simulink model "model_AllInOne1 (1)"  (R2013a)
settings: Solver=ode45  StartTime=0.0  StopTime=400  RelTol=1e-3
undefined symbols (not defined in the file or in its folder): generateDummyBeams, m, s
libraries: test_library x15, aerolib6dofsys x2, aerolibtransform2 x1, aerolibutil x1, aerolibconvert2 x1, falter_library x1, vrlib x1
(part 1 of 2)
settings Model: Creator=elm  LastModifiedBy=alim
settings DataIOCC: SignalLoggingSaveFormat=ModelDataLogs  SaveOutput=off  SignalLogging=off  DSMLogging=off  SaveTime=off
settings OptimizationCC: ExpressionDepthLimit=2147483647  EfficientMapNaN2IntZero=off
settings DebuggingCC: FcnCallInpInsideContextMsg=UseLocalSettings
settings HardwareCC: TargetBitPerLong=64  TargetBitPerPointer=64  TargetIntDivRoundTo=Zero  TargetEndianess=LittleEndian  TargetWordSize=64  TargetHWDeviceType=MATLAB Host  ProdEqTarget=off
settings SFSimCC: SimParseCustomCode=off
settings CodeAppCC: MaxIdLength=128
settings GRTTargetCC: CombineOutputUpdateFcns=off  GRTInterface=on

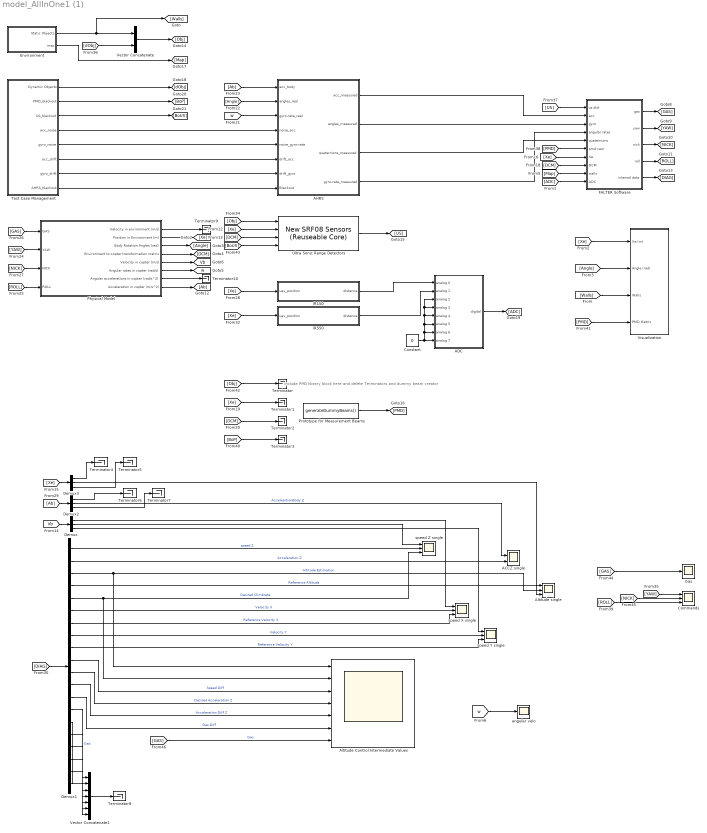
== system model_AllInOne1 (1) ==
  note: include PMD library block  here and delete Terminators
      | and dummy beam creator
  ACCZ single : Scope  NumInputPorts=2
      settings: ShowLegends=on  TimeRange=5  YMin=-9.9~9.7331  YMax=-8.7~9.7343  SaveName=ScopeData4  SampleInput=on
  ADC : Subsystem
  AHRS : Subsystem
  Altitude Control Intermediate Values : Scope  NumInputPorts=7
      settings: ShowLegends=on  TimeRange=20  YMin=0.1~-0.2~-0.9~-0.5~-0.4~-0.00015~0  YMax=1.3~0.5~0.5~0.3~0.3~0.00015~150  SaveName=ScopeData16  SampleInput=on
  Altitude single : Scope  NumInputPorts=3
      settings: TimeRange=15  YMin=0.1~0.1~0  YMax=1.3~1.3~1  SaveName=ScopeData7  SampleInput=on
  Commands : Scope  NumInputPorts=3
      settings: YMin=0~0.1~0  YMax=3.25~0.8~1  SaveName=ScopeData32  SampleInput=on
  Constant : Constant  Value=0
  Demux : Demux  Outputs=3
  Demux1 : Demux  Outputs=20
  Demux2 : Demux  Outputs=3
  Demux3 : Demux  Outputs=3
  Environment : Subsystem
  FALTER Software : Subsystem
  Gas : Scope
      settings: TimeRange=18  YMin=0  YMax=300  SaveName=ScopeData31  SampleInput=on
  IR150 : Subsystem
  IR550 : Subsystem
  Physical Model : Subsystem
  Prototype for Measurement Beams : Constant  Value=generateDummyBeams()  OutDataTypeStr=single
  Terminator{,1..10} (11 alike) : Terminator
  Test Case Management : Subsystem
  "Ultra Sonic Range Detectors " : falter_library/New SRF08 Sensors  (Reuseable Core)  a=[0.1 0 0 0 -1 0; 0 0.12 -0.07 0 -1 0; 0 0.12 0.07 0 0 1; 0 0 0.21 1 0 0; 0.07 0.12 0 1 0 0; 0 0 -0.21 1 0 0; -0.07 0.12 0 -1 0 0; 0 0.12 0 0 1 0]  t=0.05
  Vector Concatenate : Concatenate  Mode=Multidimensional array
  Vector Concatenate1 : Concatenate  NumInputs=7  Mode=Multidimensional array
  Visualization : Subsystem
  angular velo : Scope
      settings: TimeRange=7.5  YMin=-0.85  YMax=0  SaveName=ScopeData24  SampleInput=on
  speed X single : Scope  NumInputPorts=3
      settings: TimeRange=5  YMin=-0.05~-0.025~0  YMax=0.175~0.15~0.3  SaveName=ScopeData14  SampleInput=on
  speed Y single : Scope  NumInputPorts=3
      settings: YMin=0~-5~-5  YMax=10~5~5  SaveName=ScopeData25  SampleInput=on
  speed Z single : Scope  NumInputPorts=3
      settings: TimeRange=18  YMin=-5~-5~-0.2  YMax=5~5~0.2  SaveName=ScopeData5  SampleInput=on
  tag scope: Vb=global, w=global
  wires:
  [Walls] -> Visualization/3(Walls)
  [Xe] -> Visualization/1(Xe (m))
  [Angle] -> Visualization/2(Angle (rad))
  Environment/1(Static Objects) -> Vector Concatenate/1, [Walls]
  FALTER Software/1(gas) -> [GAS]
  FALTER Software/2("yaw ") -> [YAW]
  FALTER Software/3(nick) -> [NICK]
  FALTER Software/4(roll) -> [ROLL]
  Physical Model/1(Velocity in environment (m/s)) -> Terminator9/1
  Physical Model/2(Position in Environment (m)) -> [Xe]
  [Xe] -> "Ultra Sonic Range Detectors "/2
  Physical Model/7(Angular accelerations in copter (rad/s^2)) -> Terminator10/1
  Physical Model/5(Velocity in copter (m/s)) -> [Vb]
  Physical Model/4(Environment to copter transformation matrix) -> [DCM]
  Physical Model/3(Body Rotation Angles (rad)) -> [Angle]
  Physical Model/8(Acceleration in copter (m/s^2)) -> [Ab]
  [YAW] -> Physical Model/2(YAW)
  [NICK] -> Physical Model/3(NICK)
  [ROLL] -> Physical Model/4(ROLL)
  [DCM] -> "Ultra Sonic Range Detectors "/3
  Vector Concatenate/1 -> [Obj]
  [Obj] -> Terminator/1
  FALTER Software/5(internal data) -> [DIAG]
  Test Case Management/1(Dynamic Objects) -> [dObj]
  [PMD] -> Visualization/4(PMD Matrix)
  [Obj] -> "Ultra Sonic Range Detectors "/1
  [dObj] -> Vector Concatenate/2
  Test Case Management/3(US_blackout) -> [BoUS]
  Test Case Management/2(PMD_blackout) -> [BoP]
  [BoUS] -> "Ultra Sonic Range Detectors "/4
  "Ultra Sonic Range Detectors "/1 -> [US]
  [DIAG] -> Demux1/1
  [Ab] -> Demux2/1
  Demux1/9 -> speed Y single/3  "Reference Velocity Y"
  Demux1/7 -> speed X single/3  "Reference Velocity X"
  Demux1/8 -> speed Y single/2  "Velocity Y"
  [Xe] -> Demux3/1
  [Vb] -> Demux/1
  Demux1/1 -> speed Z single/2  "speed Z"
  Demux1/3 -> Altitude single/2, Altitude Control Intermediate Values/1  "Altitude Estimation"
  Demux1/4 -> Altitude single/3  "Reference Altitude"
  Demux1/2 -> ACCZ single/2  "Acceleration Z"
  Demux/2 -> speed Z single/1
  Demux1/6 -> speed X single/2  "Velocity X"
  Demux1/5 -> speed Z single/3, Altitude Control Intermediate Values/2  "Desired Climbrate"
  Demux/1 -> speed X single/1
  Demux/3 -> speed Y single/1
  Demux2/2 -> ACCZ single/1  "AcceleartionBody Z"
  Demux3/2 -> Altitude single/1
  [Xe] -> IR150/1(uav_position)
  [Xe] -> IR550/1(uav_position)
  [GAS] -> Gas/1
  [YAW] -> Commands/1
  [NICK] -> Commands/2
  [ROLL] -> Commands/3
  [GAS] -> Physical Model/1(GAS)
  Demux1/10 -> Altitude Control Intermediate Values/3  "Speed Diff"
  Demux1/11 -> Altitude Control Intermediate Values/4  "Desired Acceleration Z"
  Demux1/12 -> Altitude Control Intermediate Values/5  "Acceleration Diff Z"
  Demux1/13 -> Altitude Control Intermediate Values/6  "Gas Diff"
  [GAS] -> Altitude Control Intermediate Values/7  "Gas"
  Prototype for Measurement Beams/1 -> [PMD]
  [Xe] -> Terminator1/1
  [DCM] -> Terminator2/1
  [BoP] -> Terminator3/1
  Demux3/1 -> Terminator4/1
  Demux3/3 -> Terminator5/1
  Demux2/1 -> Terminator6/1
  Demux2/3 -> Terminator7/1
  Demux1/14 -> Vector Concatenate1/1  "Gas"
  Demux1/15 -> Vector Concatenate1/2
  Demux1/16 -> Vector Concatenate1/3
  Demux1/17 -> Vector Concatenate1/4
  Demux1/18 -> Vector Concatenate1/5
  Demux1/19 -> Vector Concatenate1/6
  Demux1/20 -> Vector Concatenate1/7
  Vector Concatenate1/1 -> Terminator8/1
  Environment/2(map) -> [Map]
  Physical Model/6(Angular rates in copter (rad/s)) -> [w]
  [w] -> angular velo/1
  ADC/1(digital) -> [ADC]
  [w] -> AHRS/3(gyro-rate_real)
  [Angle] -> AHRS/2(angles_real)
  [Ab] -> AHRS/1(acc_body)
  Test Case Management/8(AHRS_blackout) -> AHRS/8(Blackout)
  Test Case Management/7(gyro_drift) -> AHRS/7(drift_gyro)
  Test Case Management/6(acc_drift) -> AHRS/6(drift_acc)
  Test Case Management/5(gyro_noise) -> AHRS/5(noise_gyro-rate)
  Test Case Management/4(acc_noise) -> AHRS/4(noise_acc)
  AHRS/2(angles_measured) -> FALTER Software/3(gyro)
  [US] -> FALTER Software/1(us dist)
  AHRS/1(acc_measured) -> FALTER Software/2(acc)
  AHRS/3(quaternions_measured) -> FALTER Software/5(quaternions)
  AHRS/4(gyro-rate_measured) -> FALTER Software/4(angular rates)
  [PMD] -> FALTER Software/6(pmd cam)
  [Xe] -> FALTER Software/7(Xe)
  [DCM] -> FALTER Software/8(DCM)
  [Map] -> FALTER Software/9(walls)
  [ADC] -> FALTER Software/10(ADC)
  Constant/1 -> ADC/6(analog 5), ADC/5(analog 4), ADC/3(analog 2), ADC/4(analog 3), ADC/7(analog 6), ADC/8(analog 7)
  IR150/1(distance) -> ADC/1(analog 0)
  IR550/1(distance) -> ADC/2(analog 1)

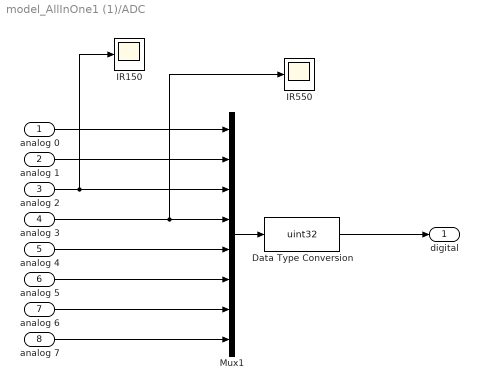
== system model_AllInOne1 (1)/ADC ==
  analog 0 : Inport
  analog 1 : Inport  Port=2
  analog 2 : Inport  Port=3
  analog 3 : Inport  Port=4
  analog 4 : Inport  Port=5
  analog 5 : Inport  Port=6
  analog 6 : Inport  Port=7
  analog 7 : Inport  Port=8
  Data Type Conversion : DataTypeConversion  OutMin=0  OutMax=1023  OutDataTypeStr=uint32
  IR150 : Scope
      settings: TimeRange=7.5  YMin=-0.85  YMax=0  SaveName=ScopeData9  SampleInput=on
  IR550 : Scope
      settings: TimeRange=7.5  YMin=-0.85  YMax=0  SaveName=ScopeData6  SampleInput=on
  Mux1 : Mux  Inputs=8
  digital : Outport
  wires:
  analog 0/1 -> Mux1/1
  analog 1/1 -> Mux1/2
  analog 2/1 -> Mux1/3, IR150/1
  analog 3/1 -> Mux1/4, IR550/1
  analog 4/1 -> Mux1/5
  analog 5/1 -> Mux1/6
  analog 6/1 -> Mux1/7
  analog 7/1 -> Mux1/8
  Mux1/1 -> Data Type Conversion/1
  Data Type Conversion/1 -> digital/1

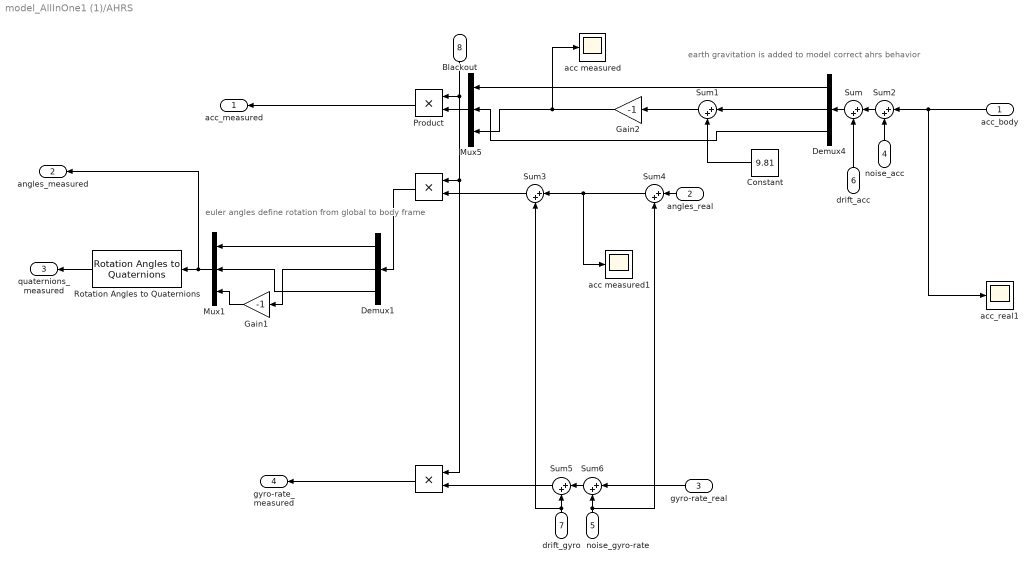
== system model_AllInOne1 (1)/AHRS ==
  note: earth gravitation is added to model correct
      | ahrs behavior
  note: euler angles define rotation
      | from global to body frame
  acc_body : Inport
  angles_real : Inport  Port=2
  gyro-rate_real : Inport  Port=3
  noise_acc : Inport  Port=4
  noise_gyro-rate : Inport  Port=5
  drift_acc : Inport  Port=6
  drift_gyro : Inport  Port=7
  Blackout : Inport  Port=8
  " " : Product  RndMeth=Zero
  "   " : Product  RndMeth=Zero
  Constant : Constant  Value=9.81
  Demux1 : Demux  Outputs=3
  Demux4 : Demux  Outputs=3
  Gain1 : Gain  Gain=-1
  Gain2 : Gain  Gain=-1
  Mux1 : Mux  Inputs=3
  Mux5 : Mux  Inputs=3
  Product : Product  RndMeth=Zero
  Rotation Angles to Quaternions : aerolibtransform2/Rotation Angles to Quaternions  rotationOrder=XYZ
  Sum{,1..6} (7 alike) : Sum  Inputs=|++
  acc measured : Scope
      settings: TimeRange=7.5  YMin=-11  YMax=-5  SampleInput=on
  acc measured1 : Scope
      settings: TimeRange=7.5  YMin=-11  YMax=-5  SaveName=ScopeData18  SampleInput=on
  acc_real1 : Scope
      settings: TimeRange=7.5  YMin=-0.85  YMax=0  SampleInput=on
  acc_measured : Outport
  angles_measured : Outport  Port=2
  quaternions_measured : Outport  Port=3
  gyro-rate_measured : Outport  Port=4
  wires:
  Demux4/1 -> Mux5/1
  " "/1 -> Demux1/1
  Sum/1 -> Demux4/1
  Sum2/1 -> Sum/1
  acc_body/1 -> Sum2/1, acc_real1/1
  noise_acc/1 -> Sum2/2
  drift_acc/1 -> Sum/2
  Mux5/1 -> Product/2
  Blackout/1 -> Product/1, " "/1, "   "/1
  Product/1 -> acc_measured/1
  Sum4/1 -> Sum3/1, acc measured1/1
  Sum3/1 -> " "/2
  angles_real/1 -> Sum4/1
  Sum6/1 -> Sum5/1
  "   "/1 -> gyro-rate_measured/1
  Sum5/1 -> "   "/2
  gyro-rate_real/1 -> Sum6/1
  drift_gyro/1 -> Sum5/2, Sum3/2
  noise_gyro-rate/1 -> Sum4/2, Sum6/2
  Rotation Angles to Quaternions/1 -> quaternions_measured/1
  Mux1/1 -> Rotation Angles to Quaternions/1, angles_measured/1
  Demux1/1 -> Mux1/1
  Demux4/2 -> Sum1/1
  Sum1/1 -> Gain2/1
  Constant/1 -> Sum1/2
  Gain2/1 -> Mux5/3, acc measured/1
  Demux4/3 -> Mux5/2
  Gain1/1 -> Mux1/3
  Demux1/3 -> Mux1/2
  Demux1/2 -> Gain1/1

== system model_AllInOne1 (1)/Environment ==
  note: basic walls for particle filter
  Terminator9 : Terminator
  environment model : Constant  RequirementInfo={}  Value=|
      | [
      |    -28     0   -16    10     0     0     0     0    32;
      |    -18     0    -5    36     0     0     0     0    10;
      |     18     0   -16    10     0     0     0     0    32;
      |     15     0     1     0     2     0     3     0     0;
      |      8     0     1     0     2     0     6     0     0;
      |      4     0     1     0     2     0     3     0     0;
      |      1     0     1     0     2     0     2     0     0;
      |     -2     0     1     0     2     0     2     0     0;
      |     -5     0     1     0     2     0     2     0     0;
      |     -8     0     1     0     2     0     3     0     0;
      |    -16     0     1     0     2     0     6     0     0;
      |    -18     0     1     0     2     0     1     0     0;
      |     15     0    -1     0     2     0     3     0     0;
      |      8     0    -1     0     2     0     6     0     0;
      |      4     0    -1     0     2     0     3     0     0;
      |      1     0    -1     0     2     0     2     0     0;
      |     -2     0    -1     0     2     0     2     0     0;
      |     -5     0    -1     0     2     0     2     0     0;
      |     -9     0    -1     0     2     0     3     0     0;
      |    -16     0    -1     0     2     0     6     0     0;
      |    -18     0    -1     0     2     0     1     0     0;
      |     10     0     5     0     2     0     0     0    -4;
      |      5     0     5     0     2     0     0     0    -4;
      |      2     0     5     0     2     0     0     0    -4;
      |     -1     0     5     0     2     0     0     0    -4;
      |     -4     0     5     0     2     0     0     0    -4;
      |     -7     0     5     0     2     0     0     0    -4;
      |    -12     0     5     0     2     0     0     0    -4;
      |     10     0    -5     0     2     0     0     0     4;
      |      5     0    -5     0     2     0     0     0     4,
      |      2     0    -5     0     2     0     0     0     4;
      |     -1     0    -5     0     2     0     0     0     4;
      |     -4     0    -5     0     2     0     0     0     4;
      |     -7     0    -5     0     2     0     0     0     4;
      |    -12     0    -5     0     2     0     0     0     4;
      |    -18     0     5     0     2     0    36     0     0;
      |    -18     0    -5     0     2     0    36     0     0;
      |     22     0   -11     0     2     0     0     0    -5;
      |     22     0    -8     0     2     0     0     0    -2;
      |     22     0    -5     0     2     0     0     0    -2;
      |     22     0    -1     0     2     0     0     0    -3;
      |     22     0     6     0     2     0     0     0    -5;
      |     22     0     8     0     2     0     0     0    -1;
      |     22     0    11     0     2     0     0     0    -2;
      |     22     0    16     0     2     0     0     0    -4;
      |     18     0    -9     0     2     0     4     0     0;
      |     18     0    -5     0     2     0     4     0     0;
      |     18     0    -1     0     2     0     4     0     0;
      |     18     0     1     0     2     0     4     0     0;
      |     18     0     7     0     2     0     4     0     0;
      |     18     0     9     0     2     0     4     0     0;
      |    -22     0   -11     0     2     0     0     0    -5;
      |    -22     0    -8     0     2     0     0     0    -2;
      |    -22     0    -5     0     2     0     0     0    -2;
      |    -22     0    -1     0     2     0     0     0    -3;
      |    -22     0     6     0     2     0     0     0    -5;
      |    -22     0     8     0     2     0     0     0    -1;
      |    -22     0    11     0     2     0     0     0    -2;
      |    -22     0    16     0     2     0     0     0    -4;
      |    -18     0    16     0     2     0     0     0   -15;
      |     18     0    16     0     2     0     0     0   -15;
      |     18     0   -16     0     2     0     0     0    15;
      |    -18     0   -16     0     2     0     0     0    15;
      |    -18     0    -9     0     2     0    -4     0     0;
      |    -18     0    -5     0     2     0    -4     0     0;
      |    -18     0    -1     0     2     0    -4     0     0;
      |    -18     0     1     0     2     0    -4     0     0;
      |    -18     0     7     0     2     0    -4     0     0;
      |    -18     0     9     0     2     0    -4     0     0;
      |     24     0   -14     0     2     0     0     0    -2;
      |     24     0    -6     0     2     0     0     0    -5;
      |     24     0    -4     0     2     0     0     0    -1;
      |     24     0    -1     0     2     0     0     0    -2;
      |     24     0     3     0     2     0     0     0    -2;
      |     24     0     5     0     2     0     0     0    -1;
      |     24     0    11     0     2     0     0     0    -5;
      |     24     0    16     0     2     0     0     0    -3;
      |     28     0   -12     0     2     0    -4     0     0;
      |     28     0    -8     0     2     0    -4     0     0;
      |     28     0    -5     0     2     0    -4     0     0;
      |     28     0    -1     0     2     0    -4     0     0;
      |     28     0     1     0     2     0    -4     0     0;
      |     28     0     5     0     2     0    -4     0     0;
      |     28     0     8     0     2     0    -4     0     0;
      |     28     0    12     0     2     0    -4     0     0;
      |    -24     0   -14     0     2     0     0     0    -2;
      |    -24     0    -6     0     2     0     0     0    -5;
      |    -24     0    -4     0     2     0     0     0    -1;
      |    -24     0    -1     0     2     0     0     0    -2;
      |    -24     0     3     0     2     0     0     0    -2;
      |    -24     0     5     0     2     0     0     0    -1;
      |    -24     0    11     0     2     0     0     0    -5;
      |    -24     0    16     0     2     0     0     0    -3;
      |    -28     0   -12     0     2     0     4     0     0;
      |    -28     0    -8     0     2     0     4     0     0;
      |    -28     0    -5     0     2     0     4     0     0;
      |    -28     0    -1     0     2     0     4     0     0;
      |    -28     0     1     0     2     0     4     0     0;
      |    -28     0     5     0     2     0     4     0     0;
      |    -28     0     8     0     2     0     4     0     0;
      |    -28     0    12     0     2     0     4     0     0;
      |    -28     0   -16     0     2     0    10     0     0;
      |    -28     0    16     0     2     0    10     0     0;
      |     28     0    16     0     2     0   -10     0     0;
      |     28     0   -16     0     2     0   -10     0     0;
      |     28     0   -16     0     2     0     0     0    32;
      |    -28     0   -16     0     2     0     0     0    32;
      | ]
  environment model1 : Constant  RequirementInfo={} %GIDa_a9006805_dc84_4529_b501_c6e675685754  Value=|
      | [
      |    -28     0   -16    10     0     0     0     0    32;
      |    -18     0    -5    36     0     0     0     0    10;
      |     18     0   -16    10     0     0     0     0    32;
      |    -24     0     1     0     2     0    -4     0     0;
      |    -24     0    -1     0     2     0    -4     0     0;
      |    -24     0    -1     0     2     0     0     0   -15;
      |    -22     0    -1     0     2     0     0     0   -15;
      |    -24     0     1     0     2     0     0     0    15;
      |    -22     0     1     0     2     0     0     0    15;
      |     22     0     1     0     2     0   -44     0     0;
      |     22     0    -1     0     2     0   -44     0     0;
      |     22     0    -1     0     2     0     0     0   -15;
      |     24     0    -1     0     2     0     0     0   -15;
      |     24     0    -1     0     2     0     4     0     0;
      |     24     0     1     0     2     0     4     0     0;
      |     22     0     1     0     2     0     0     0    15;
      |     24     0     1     0     2     0     0     0    15;
      |    -28     0   -16     0     2     0     0     0    32;
      |    -18     0   -16     0     2     0   -10     0     0;
      |    -18     0    16     0     2     0   -10     0     0;
      |    -18     0     5     0     2     0     0     0    11;
      |    -18     0    -5     0     2     0     0     0   -11;
      |     18     0     5     0     2     0   -36     0     0;
      |     18     0    -5     0     2     0   -36     0     0;
      |     18     0   -16     0     2     0     0     0    11;
      |     18     0    16     0     2     0     0     0   -11;
      |     28     0   -16     0     2     0   -10     0     0;
      |     28     0    16     0     2     0   -10     0     0;
      |     28     0    16     0     2     0     0     0   -32;
      |     0      0    0      0     0     0     0     0     0;
      |     0      0    0      0     0     0     0     0     0;
      |     0      0    0      0     0     0     0     0     0;
      |     0      0    0      0     0     0     0     0     0;
      |     0      0    0      0     0     0     0     0     0;
      |     0      0    0      0     0     0     0     0     0;
      |     0      0    0      0     0     0     0     0     0;
      |     0      0    0      0     0     0     0     0     0;
      |     0      0    0      0     0     0     0     0     0;
      |     0      0    0      0     0     0     0     0     0;
      |     0      0    0      0     0     0     0     0     0;
      |     0      0    0      0     0     0     0     0     0;
      |     0      0    0      0     0     0     0     0     0;
      |     0      0    0      0     0     0     0     0     0;
      |     0      0    0      0     0     0     0     0     0;
      |     0      0    0      0     0     0     0     0     0;
      |     0      0    0      0     0     0     0     0     0;
      |     0      0    0      0     0     0     0     0     0;
      | ]
  Static Objects : Outport
  map : Outport  Port=2
  wires:
  environment model1/1 -> map/1, Static Objects/1
  environment model/1 -> Terminator9/1

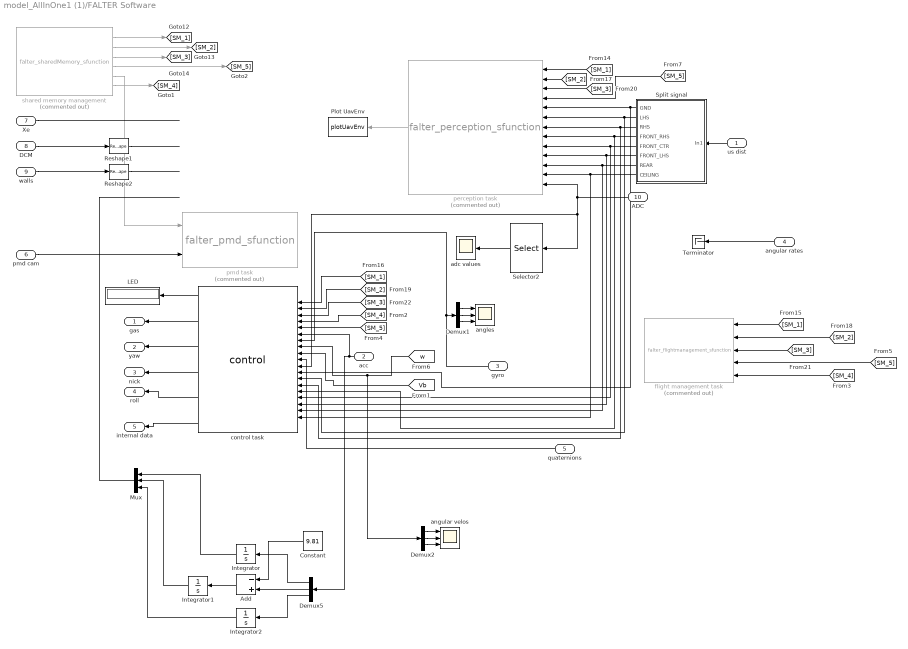
== system model_AllInOne1 (1)/FALTER Software ==
  us dist : Inport
  acc : Inport  Port=2
  gyro : Inport  Port=3
  angular rates : Inport  Port=4
  quaternions : Inport  Port=5
  pmd cam : Inport  Port=6
  Xe : Inport  Port=7
  DCM : Inport  Port=8
  walls : Inport  Port=9
  ADC : Inport  Port=10  OutDataTypeStr=uint32
  Add : Sum  Inputs=-+
  Constant : Constant  Value=9.81
  Demux1 : Demux  Outputs=3
  Demux2 : Demux  Outputs=3
  Demux5 : Demux  Outputs=3
  Integrator : Integrator
  Integrator1 : Integrator
  Integrator2 : Integrator
  LED : Display
  Mux : Mux  Inputs=3
  Plot UavEnv : MATLABFcn  MATLABFcn=plotUavEnv  OutputDimensions=0  SampleTime=0.05
  Reshape1 : Reshape  OutputDimensionality=Row vector (2-D)
  Reshape2 : Reshape  OutputDimensionality=Row vector (2-D)
  Selector2 : Selector  IndexMode=Zero-based  InputPortWidth=8  IndexOptions=Index vector (dialog)  Indices=[2 3 4]  OutputSizes=1
  Split signal : Subsystem
  Terminator : Terminator
  adc values : Scope
      settings: TimeRange=7.5  YMin=-0.85  YMax=0  SaveName=ScopeData28  SampleInput=on
  angles : Scope  NumInputPorts=3
      settings: TimeRange=7.5  YMin=-0.85~-5~-5  YMax=0~5~5  SaveName=ScopeData17  SampleInput=on
  angular velos : Scope  NumInputPorts=3
      settings: TimeRange=7.5  YMin=-0.85~-5~-5  YMax=0~5~5  SaveName=ScopeData26  SampleInput=on
  control task : S-Function  FunctionName=control  EnableBusSupport=off
      mask Display:
      | port_label('input',1,'obstacle flags')
      | port_label('input',2,'position data')
      | port_label('input',3,'uav env data')
      | port_label('input',4,'ctrl ref')
      | port_label('input',5,'errors')
      | 
      | port_label('input',6,'acc')
      | port_label('input',7,'gyro')
      | port_label('input',8,'rotational speed')
      | port_label('input',9,'magic speed')
      | port_label('input',10,'quaternions')
      | port_label('input',11,'adc')
      | port_label('input',12,'srf_gnd')
      | port_label('input',13,'srf_lhs')
      | port_label('input',14,'srf_rhs')
      | port_label('input',15,'srf_front_rhs')
      | port_label('input',16,'srf_front_ctr')
      | port_label('input',17,'srf_front_lhs')
      | port_label('input',18,'srf_rear')
      | port_label('input',19,'srf_ceiling')
      | 
      | port_label('output',1,'led')
      | port_label('output',2,'gas')
      | port_label('output',3,'yaw')
      | port_label('output',4,'nick')
      | port_label('output',5,'roll')
  flight management task : S-Function  Commented=on  FunctionName=falter_flightmanagement_sfunction  EnableBusSupport=off
      mask Display:
      | port_label('input',1,'obstacle flags')
      | port_label('input',2,'position data')
      | port_label('input',3,'uav env')
      | port_label('input',4,'errors')
      | 
      | port_label('input',5,'ctrl ref')
  perception task : S-Function  Commented=on  FunctionName=falter_perception_sfunction  EnableBusSupport=off
      mask Display:
      | port_label('input',1,'obstacle flags')
      | port_label('input',2,'position data')
      | port_label('input',3,'uav env')
      | port_label('input',4,'errors')
      | 
      | port_label('input',5,'SRF_GND')
      | port_label('input',6,'SRF_LHS')
      | port_label('input',7,'SRF_RHS')
      | port_label('input',8,'SRF_FRONT_RHS')
      | port_label('input',9,'SRF_FRONT_CTR')
      | port_label('input',10,'SRF_FRONT_LHS')
      | port_label('input',11,'SRF_REAR')
      | port_label('input',12,'SRF_CEILING')
      | port_label('input',13,'ADC')
      | 
      | port_label('output',1,'UAV Environment')
  pmd task : S-Function  Commented=on  FunctionName=falter_pmd_sfunction  EnableBusSupport=off
      mask Display:
      | port_label('input',1,'pmd_data (shm)')
      | port_label('input',2,'pmd distances')
  shared memory management : S-Function  Commented=on  FunctionName=falter_sharedMemory_sfunction  EnableBusSupport=off
      mask Display:
      | port_label('output', 1, 'obstacle flags')
      | port_label('output', 2, 'position data')
      | port_label('output', 3, 'uav env')
      | port_label('output', 4, 'errors')
      | port_label('output', 5, 'pmd data')
      | port_label('output', 6, 'ctrl ref')
      | 
      | disp('SHM')
  gas : Outport
  "yaw " : Outport  Port=2
  nick : Outport  Port=3
  roll : Outport  Port=4
  internal data : Outport  Port=5
  wires:
  control task/1 -> LED/1
  [SM_1] -> perception task/1
  [SM_1] -> flight management task/1
  [SM_1] -> control task/1
  [SM_2] -> perception task/2
  [SM_2] -> flight management task/2
  [SM_2] -> control task/2
  [SM_3] -> perception task/3
  [SM_3] -> flight management task/3
  [SM_3] -> control task/3
  shared memory management/3 -> [SM_3]
  shared memory management/2 -> [SM_2]
  shared memory management/1 -> [SM_1]
  Split signal/1(GND) -> perception task/5, control task/12
  Split signal/2(LHS) -> control task/13, perception task/6
  Split signal/3(RHS) -> control task/14, perception task/7
  Split signal/4(FRONT_RHS) -> control task/15, perception task/8
  Split signal/5(FRONT_CTR) -> control task/16, perception task/9
  Split signal/6(FRONT_LHS) -> control task/17, perception task/10
  Split signal/7(REAR) -> control task/18, perception task/11
  Split signal/8(CEILING) -> control task/19, perception task/12
  gyro/1 -> control task/7, Demux1/1
  acc/1 -> Demux5/1, control task/6
  us dist/1 -> Split signal/1(In1)
  perception task/1 -> Plot UavEnv/1
  shared memory management/5 -> pmd task/1
  pmd cam/1 -> pmd task/2
  Xe/1 -> ?
  Reshape1/1 -> ?
  DCM/1 -> Reshape1/1
  walls/1 -> Reshape2/1
  Reshape2/1 -> ?
  Demux5/1 -> Integrator/1
  Demux5/3 -> Integrator2/1
  Constant/1 -> Add/1
  Demux5/2 -> Add/2
  Add/1 -> Integrator1/1
  Integrator/1 -> Mux/1
  Integrator1/1 -> Mux/2
  Integrator2/1 -> Mux/3
  Mux/1 -> ?
  [w] -> control task/8, Demux2/1
  [Vb] -> control task/9
  quaternions/1 -> control task/10
  ADC/1 -> perception task/13, Selector2/1, control task/11
  shared memory management/6 -> [SM_4]
  [SM_4] -> control task/4
  [SM_4] -> flight management task/5
  control task/2 -> gas/1
  control task/3 -> "yaw "/1
  control task/4 -> nick/1
  control task/5 -> roll/1
  control task/6 -> internal data/1
  Demux1/1 -> angles/1
  Demux1/2 -> angles/2
  Demux1/3 -> angles/3
  Demux2/1 -> angular velos/1
  Demux2/2 -> angular velos/2
  Demux2/3 -> angular velos/3
  angular rates/1 -> Terminator/1
  Selector2/1 -> adc values/1
  shared memory management/4 -> [SM_5]
  [SM_5] -> control task/5
  [SM_5] -> flight management task/4
  [SM_5] -> perception task/4

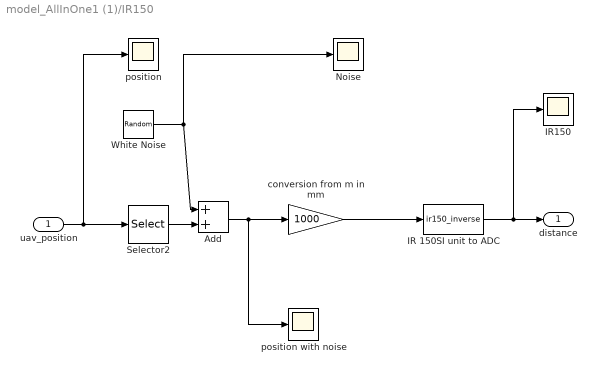
== system model_AllInOne1 (1)/IR150 ==
  uav_position : Inport
  Add : Sum
  IR 150SI unit to ADC : MATLABFcn  MATLABFcn=ir150_inverse
  IR150 : Scope
      settings: TimeRange=7.5  YMin=-0.85  YMax=0  SaveName=ScopeData15  SampleInput=on
  Noise : Scope
      settings: TimeRange=7.5  YMin=-0.85  YMax=0  SaveName=ScopeData10  SampleInput=on
  Selector2 : Selector  IndexMode=Zero-based  InputPortWidth=3  IndexOptions=Index vector (dialog)  Indices=[1]  OutputSizes=1
  White Noise : RandomNumber  DisableCoverage=on  Variance=0.0001  Seed=234987234  SampleTime=0
  conversion from m in mm : Gain  Gain=1000
  position : Scope
      settings: TimeRange=7.5  YMin=-0.85  YMax=0  SaveName=ScopeData11  SampleInput=on
  position with noise : Scope
      settings: TimeRange=7.5  YMin=-0.85  YMax=0  SaveName=ScopeData12  SampleInput=on
  distance : Outport
  wires:
  White Noise/1 -> Add/1, Noise/1
  Add/1 -> position with noise/1, conversion from m in mm/1
  IR 150SI unit to ADC/1 -> distance/1, IR150/1
  uav_position/1 -> Selector2/1, position/1
  Selector2/1 -> Add/2
  conversion from m in mm/1 -> IR 150SI unit to ADC/1

== system model_AllInOne1 (1)/IR550 ==
  uav_position : Inport
  Add : Sum
  IR 550 SI unit to ADC : MATLABFcn  MATLABFcn=ir550_inverse
  Noise : Scope
      settings: TimeRange=7.5  YMin=-0.85  YMax=0  SaveName=ScopeData29  SampleInput=on
  Selector2 : Selector  IndexMode=Zero-based  InputPortWidth=3  IndexOptions=Index vector (dialog)  Indices=[1]  OutputSizes=1
  White Noise : RandomNumber  DisableCoverage=on  Variance=0.0001  Seed=234987234  SampleTime=0
  conversion from m in mm : Gain  Gain=1000
  position with noise : Scope
      settings: TimeRange=7.5  YMin=-0.85  YMax=0  SaveName=ScopeData30  SampleInput=on
  distance : Outport
  wires:
  Add/1 -> conversion from m in mm/1, position with noise/1
  IR 550 SI unit to ADC/1 -> distance/1
  uav_position/1 -> Selector2/1
  Selector2/1 -> Add/2
  conversion from m in mm/1 -> IR 550 SI unit to ADC/1
  White Noise/1 -> Add/1, Noise/1

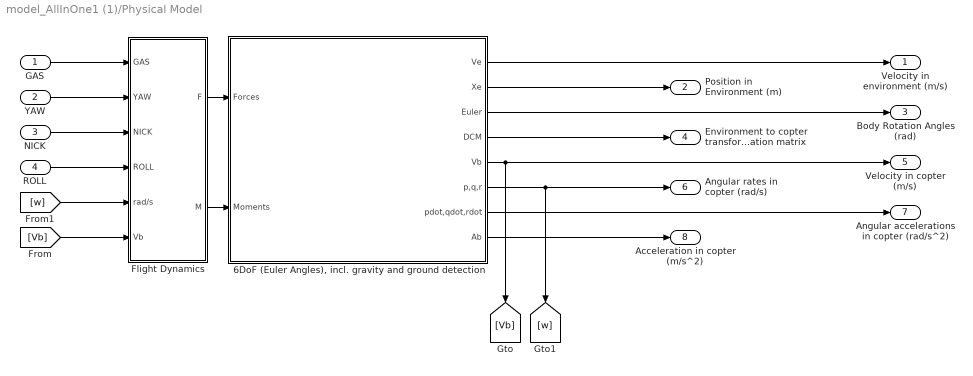
== system model_AllInOne1 (1)/Physical Model ==
  GAS : Inport
  YAW : Inport  Port=2
  NICK : Inport  Port=3
  ROLL : Inport  Port=4
  "6DoF (Euler Angles), incl. gravity and ground detection" : Subsystem  mask(6DoF EoM (Body Axis)){units=Metric (MKS), mtype=Fixed, rep=Euler Angles, xme_0=[-23 0.12 -4], Vm_0=[0 0 0], eul_0=[0 (-pi*1)/2 0], pm_0=[0 0 0], mass_0=1.5, mass_e=0.5, mass_f=2.0, inertia=eye(3), inertia_e=eye(3), inertia_f=2*eye(3), k_quat=1.0}
      mask prompts: mtype "Mass type:"; rep "Representation:"; xme_0 "Initial position in inertial axes [Xe,Ye,Ze]:"; Vm_0 "Initial velocity in body axes [U,v,w]:"; eul_0 "Initial Euler orientation [roll, pitch, yaw]:"; pm_0 "Initial body rotation rates [p,q,r]:"; mass_0 "Initial mass:"; mass_e "Empty mass:"; mass_f "Full mass:"; inertia_e "Empty inertia matrix:"; inertia_f "Full inertia matrix:"; k_quat "Gain for quaternion normalization:"
      mask help: Integrate the six-degrees-of-freedom equations of motion in body axis.
      mask Help: eval('asbhelp(''sixdof_euler_angles'')');
      mask TypeOptions units: Metric (MKS) | English (Velocity in ft/s) | English (Velocity in kts)
      mask TypeOptions mtype: Fixed | Simple Variable | Custom Variable
      mask Callback mtype: aeroicon('aeroblk6dofbody');
      mask TypeOptions rep: Euler Angles | Quaternion
      mask Callback rep: aeroicon('aeroblk6dofbody');
  Flight Dynamics : Subsystem
  Velocity in environment (m/s) : Outport
  Position in Environment (m) : Outport  Port=2
  Body Rotation Angles (rad) : Outport  Port=3
  Environment to copter transformation matrix : Outport  Port=4
  Velocity in copter (m/s) : Outport  Port=5
  Angular rates in copter (rad/s) : Outport  Port=6
  Angular accelerations in copter (rad/s^2) : Outport  Port=7
  Acceleration in copter (m/s^2) : Outport  Port=8
  wires:
  Flight Dynamics/1(F) -> "6DoF (Euler Angles), incl. gravity and ground detection"/1(Forces)
  Flight Dynamics/2(M) -> "6DoF (Euler Angles), incl. gravity and ground detection"/2(Moments)
  "6DoF (Euler Angles), incl. gravity and ground detection"/1(Ve) -> Velocity in environment (m/s)/1
  "6DoF (Euler Angles), incl. gravity and ground detection"/2(Xe) -> Position in Environment (m)/1
  GAS/1 -> Flight Dynamics/1(GAS)
  YAW/1 -> Flight Dynamics/2(YAW)
  NICK/1 -> Flight Dynamics/3(NICK)
  "6DoF (Euler Angles), incl. gravity and ground detection"/4(DCM) -> Environment to copter transformation matrix/1
  ROLL/1 -> Flight Dynamics/4(ROLL)
  "6DoF (Euler Angles), incl. gravity and ground detection"/6(p,q,r) -> Angular rates in copter (rad/s)/1, [w]
  "6DoF (Euler Angles), incl. gravity and ground detection"/7(pdot,qdot,rdot) -> Angular accelerations in copter (rad/s^2)/1
  [Vb] -> Flight Dynamics/6(Vb)
  [w] -> Flight Dynamics/5(rad/s)
  "6DoF (Euler Angles), incl. gravity and ground detection"/3(Euler) -> Body Rotation Angles (rad)/1
  "6DoF (Euler Angles), incl. gravity and ground detection"/8(Ab) -> Acceleration in copter (m/s^2)/1
  "6DoF (Euler Angles), incl. gravity and ground detection"/5(Vb) -> Velocity in copter (m/s)/1, [Vb]

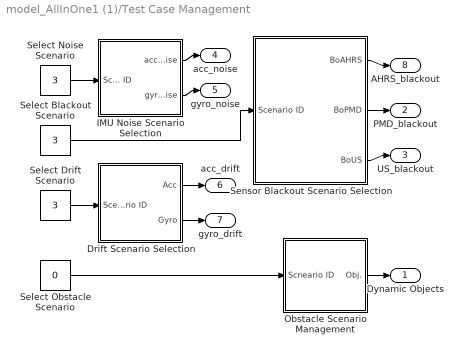
== system model_AllInOne1 (1)/Test Case Management ==
  Drift Scenario Selection : Subsystem
  IMU Noise Scenario Selection : Subsystem
  Obstacle Scenario Management : Subsystem
  Select Blackout Scenario : Constant  Value=3
  Select Drift Scenario : Constant  Value=3
  Select Noise Scenario : Constant  Value=3
  Select Obstacle Scenario : Constant  Value=0
  Sensor Blackout Scenario Selection : Subsystem
  Dynamic Objects : Outport
  PMD_blackout : Outport  Port=2
  US_blackout : Outport  Port=3
  acc_noise : Outport  Port=4
  gyro_noise : Outport  Port=5
  acc_drift : Outport  Port=6
  gyro_drift : Outport  Port=7
  AHRS_blackout : Outport  Port=8
  wires:
  Obstacle Scenario Management/1(Obj.) -> Dynamic Objects/1
  Select Noise Scenario/1 -> IMU Noise Scenario Selection/1(Scenario ID)
  Select Obstacle Scenario/1 -> Obstacle Scenario Management/1(Scneario ID)
  Drift Scenario Selection/2(Gyro) -> gyro_drift/1
  Drift Scenario Selection/1(Acc) -> acc_drift/1
  Select Drift Scenario/1 -> Drift Scenario Selection/1(Scenario ID)
  IMU Noise Scenario Selection/1(acc_noise) -> acc_noise/1
  IMU Noise Scenario Selection/2(gyro_noise) -> gyro_noise/1
  Select Blackout Scenario/1 -> Sensor Blackout Scenario Selection/1(Scenario ID)
  Sensor Blackout Scenario Selection/1(BoAHRS) -> AHRS_blackout/1
  Sensor Blackout Scenario Selection/2(BoPMD) -> PMD_blackout/1
  Sensor Blackout Scenario Selection/3(BoUS) -> US_blackout/1

== system model_AllInOne1 (1)/Visualization ==
  Xe (m) : Inport
  Angle (rad) : Inport  Port=2
  Walls : Inport  Port=3
  PMD Matrix : Inport  Port=4  OutDataTypeStr=single
  3D Simulation : vrlib/VR Sink  InstantiateOnLoad=on  SampleTime=0.1  ViewEnable=on  RemoteChange=off  RemoteView=off  FieldsWritten=Falter.rotation.4.1.1.double#Falter.translation.3.1.1.double#faltercamera.orientation.4.1.1.double#faltercamera.position.3.1.1.double  WorldFileName=./3DSimulation/walls.wrl  WorldDescription=Falter  AutoView=on  VideoDimensions=[]  AllowVariableSize=off  FigureProperties="{'Position', 'Name', 'Viewpoint', 'CameraBound', 'CameraDirection', 'CameraPosition', 'CameraUpVector', 'ZoomFactor', 'Antialiasing', 'Headlight', 'Lighting', 'NavPanel', 'StatusBar', 'ToolBar', 'Textures', 'Transparency', 'Triad', 'Wireframe', 'NavZones', 'NavMode', 'NavSpeed', 'CaptureFileFormat', 'CaptureFileName', 'Record2DCompressMethod', 'Record2DCompressQuality', 'Record2D', 'Record2DFileName', 'Record2DFPS'; [7.6000000000000000e+01   1.1600000000000000e+02   5.7600000000000000e+02   3.8000000000000000e+02], 'Falter', 'here', 'on', [0.0000000000000000e+00   0.0000000000000000e+00  -1.0000000000000000e+00], [0.0000000000000000e+00   0.0000000000000000e+00   0.0000000000000000e+00], [0.0000000000000000e+00   1.0000000000000000e+00   0.0000000000000000e+00], [1.0000000000000000e+00], 'on', 'on', 'on', 'halfbar', 'on', 'on', 'on', 'on', 'none', 'off', 'off', 'examine', 'normal', 'tif', '%f_anim_%n.tif', 'auto', [7.5000000000000000e+01], 'off', '%f_anim_%n.avi', [1.5000000000000000e+01]}"
  Plot PMD Cam Image : Subsystem
  Rotation : Subsystem
  Scope : Scope
      settings: YMin=-25  YMax=2.5  SaveName=ScopeData3
  raum.m : MATLABFcn  MATLABFcn=raum  OutputDimensions=0  Output1D=off  SampleTime=1000
  wires:
  Xe (m)/1 -> 3D Simulation/2, 3D Simulation/4, Scope/1
  Walls/1 -> raum.m/1
  Angle (rad)/1 -> Rotation/1(phi theta psi 3x1)
  PMD Matrix/1 -> Plot PMD Cam Image/1(In1)
  Rotation/1(falter rotation) -> 3D Simulation/1
  Rotation/2(faltercamera rotation) -> 3D Simulation/3

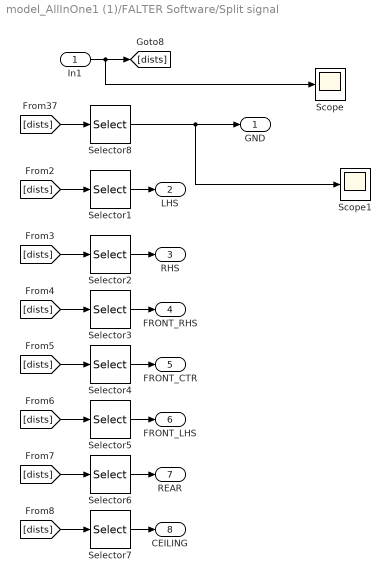
== system model_AllInOne1 (1)/FALTER Software/Split signal ==
  In1 : Inport
  Scope : Scope
      settings: YMin=-5e+275  YMax=5e+274  SaveName=ScopeData13
  Scope1 : Scope
      settings: YMin=-5e+275  YMax=5e+274  SaveName=ScopeData2
  Selector1 : Selector  NumberOfDimensions=2  InputPortWidth=3  IndexOptions=Index vector (dialog),Select all  Indices=2,1  OutputSizes=1,1
  Selector2 : Selector  NumberOfDimensions=2  InputPortWidth=3  IndexOptions=Index vector (dialog),Select all  Indices=3,1  OutputSizes=1,1
  Selector3 : Selector  NumberOfDimensions=2  InputPortWidth=3  IndexOptions=Index vector (dialog),Select all  Indices=4,1  OutputSizes=1,1
  Selector4 : Selector  NumberOfDimensions=2  InputPortWidth=3  IndexOptions=Index vector (dialog),Select all  Indices=5,1  OutputSizes=1,1
  Selector5 : Selector  NumberOfDimensions=2  InputPortWidth=3  IndexOptions=Index vector (dialog),Select all  Indices=6,1  OutputSizes=1,1
  Selector6 : Selector  NumberOfDimensions=2  InputPortWidth=3  IndexOptions=Index vector (dialog),Select all  Indices=7,1  OutputSizes=1,1
  Selector7 : Selector  NumberOfDimensions=2  InputPortWidth=3  IndexOptions=Index vector (dialog),Select all  Indices=8,1  OutputSizes=1,1
  Selector8 : Selector  NumberOfDimensions=2  InputPortWidth=3  IndexOptions=Index vector (dialog),Select all  Indices=1,1  OutputSizes=1,1
  GND : Outport
  LHS : Outport  Port=2
  RHS : Outport  Port=3
  FRONT_RHS : Outport  Port=4
  FRONT_CTR : Outport  Port=5
  FRONT_LHS : Outport  Port=6
  REAR : Outport  Port=7
  CEILING : Outport  Port=8
  wires:
  Selector2/1 -> RHS/1
  Selector3/1 -> FRONT_RHS/1
  Selector4/1 -> FRONT_CTR/1
  Selector5/1 -> FRONT_LHS/1
  Selector6/1 -> REAR/1
  Selector7/1 -> CEILING/1
  Selector1/1 -> LHS/1
  Selector8/1 -> GND/1, Scope1/1
  [dists] -> Selector8/1
  [dists] -> Selector1/1
  [dists] -> Selector2/1
  [dists] -> Selector3/1
  [dists] -> Selector4/1
  [dists] -> Selector5/1
  [dists] -> Selector6/1
  [dists] -> Selector7/1
  In1/1 -> [dists], Scope/1

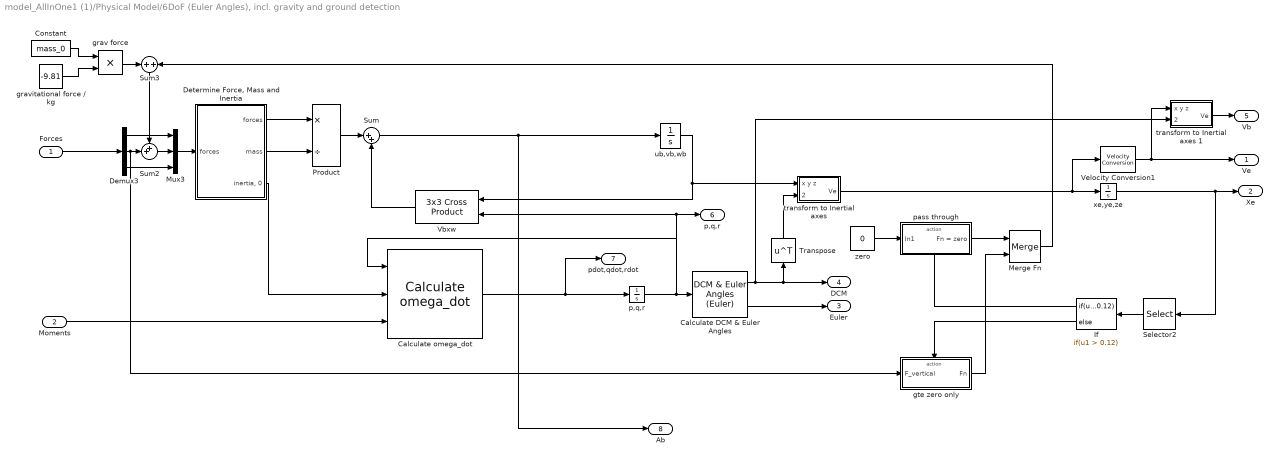
== system model_AllInOne1 (1)/Physical Model/6DoF (Euler Angles), incl. gravity and ground detection ==
  Forces : Inport
  Moments : Inport  Port=2
  Calculate DCM & Euler Angles : aerolib6dofsys/DCM & Euler Angles (Euler)  SystemSampleTime=-1
  Calculate omega_dot : aerolib6dofsys/Calculate omega_dot
  Constant : Constant  Value=mass_0  OutDataTypeStr=Inherit: Inherit via back propagation
  Demux3 : Demux  Outputs=3
  "Determine Force, Mass and Inertia" : Subsystem  TreatAsAtomicUnit=on
  If : If  IfExpression=u1 > 0.12
  Merge Fn : Merge
  Mux3 : Mux  Inputs=3
  Product : Product  Inputs=*/  SaturateOnIntegerOverflow=on  OutDataTypeStr=Inherit: Same as first input
  Selector2 : Selector  IndexMode=Zero-based  InputPortWidth=3  IndexOptions=Index vector (dialog)  Indices=[1]  OutputSizes=1
  Sum : Sum  Inputs=|++  SaturateOnIntegerOverflow=on
  Sum2 : Sum  Inputs=++|
  Sum3 : Sum  Inputs=+|+
  Transpose : Math  Operator=transpose  SaturateOnIntegerOverflow=on
  Vbxw : aerolibutil/3x3 Cross Product
  Velocity Conversion1 : aerolibconvert2/Velocity Conversion  IU=m/s  OU=m/s
  grav force : Product  RndMeth=Zero
  gravitational force / kg : Constant  Value=-9.81
  gte zero only : Subsystem  TreatAsAtomicUnit=on
  "p,q,r " : Integrator  InitialCondition=pm_0
  pass through : Subsystem  TreatAsAtomicUnit=on
  "transform to Inertial axes " : Subsystem  mask(Vector Transformation){}
      mask Display: disp('L_EB')
  transform to Inertial axes 1 : Subsystem  mask(Vector Transformation){}
      mask Display: disp('L_EB')
  ub,vb,wb : Integrator  InitialCondition=convvel(Vm_0,'m/s','m/s')
  xe,ye,ze : Integrator  InitialCondition=xme_0
  zero : Constant  Value=0
  Ve : Outport
  Xe : Outport  Port=2
  Euler : Outport  Port=3
  DCM : Outport  Port=4
  Vb : Outport  Port=5
  p,q,r : Outport  Port=6
  pdot,qdot,rdot : Outport  Port=7
  Ab : Outport  Port=8
  wires:
  Calculate omega_dot/1 -> "p,q,r "/1, pdot,qdot,rdot/1
  Transpose/1 -> "transform to Inertial axes "/2(transform coefficients)
  Calculate DCM & Euler Angles/1 -> Transpose/1, DCM/1, transform to Inertial axes 1/2(transform coefficients)
  Product/1 -> Sum/1
  Moments/1 -> Calculate omega_dot/3
  "p,q,r "/1 -> Calculate omega_dot/1, Calculate DCM & Euler Angles/1, Vbxw/2, p,q,r/1
  xe,ye,ze/1 -> Xe/1, Selector2/1
  ub,vb,wb/1 -> Vbxw/1, "transform to Inertial axes "/1(x y z)
  Calculate DCM & Euler Angles/2 -> Euler/1
  Velocity Conversion1/1 -> Ve/1, transform to Inertial axes 1/1(x y z)
  If/1 -> pass through/Action
  "transform to Inertial axes "/1(Ve) -> xe,ye,ze/1, Velocity Conversion1/1
  If/2 -> gte zero only/Action
  transform to Inertial axes 1/1(Ve) -> Vb/1
  Sum/1 -> ub,vb,wb/1, Ab/1
  Vbxw/1 -> Sum/2
  Demux3/2 -> gte zero only/1(F_vertical), Sum2/2
  Forces/1 -> Demux3/1
  Demux3/1 -> Mux3/1
  Demux3/3 -> Mux3/3
  pass through/1(Fn = zero) -> Merge Fn/1
  gte zero only/1(Fn) -> Merge Fn/2
  Merge Fn/1 -> Sum3/2
  Sum3/1 -> Sum2/1
  Sum2/1 -> Mux3/2
  Constant/1 -> grav force/1
  gravitational force / kg/1 -> grav force/2
  grav force/1 -> Sum3/1
  Selector2/1 -> If/1
  zero/1 -> pass through/1(In1)
  "Determine Force, Mass and Inertia"/1("forces ") -> Product/1
  "Determine Force, Mass and Inertia"/2(mass) -> Product/2
  "Determine Force, Mass and Inertia"/3("inertia, 0") -> Calculate omega_dot/2
  Mux3/1 -> "Determine Force, Mass and Inertia"/1(forces)

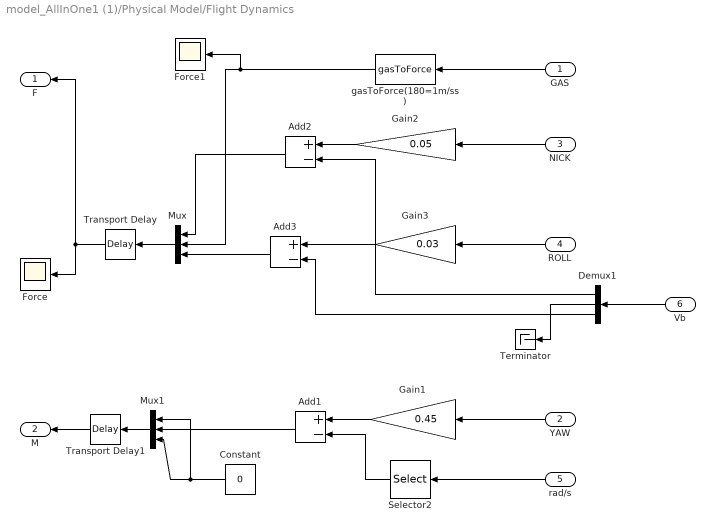
== system model_AllInOne1 (1)/Physical Model/Flight Dynamics ==
  GAS : Inport
  YAW : Inport  Port=2
  NICK : Inport  Port=3
  ROLL : Inport  Port=4
  rad/s : Inport  Port=5
  Vb : Inport  Port=6
  Add1 : Sum  Inputs=+-
  Add2 : Sum  Inputs=+-
  Add3 : Sum  Inputs=+-
  Constant : Constant  Value=0
  Demux1 : Demux  Outputs=3
  Force : Scope
      settings: YMin=-15  YMax=27.5  SaveName=ScopeData8  SampleInput=on
  Force1 : Scope
      settings: YMin=11  YMax=15.5  SaveName=ScopeData33  SampleInput=on
  Gain1 : Gain  Gain=0.45
  Gain2 : Gain  Gain=0.05
  Gain3 : Gain  Gain=0.03
  Mux : Mux  Inputs=3
  Mux1 : Mux  Inputs=3
  Selector2 : Selector  IndexMode=Zero-based  InputPortWidth=3  IndexOptions=Index vector (dialog)  Indices=[1]  OutputSizes=1
  Terminator : Terminator
  Transport Delay : TransportDelay  DelayTime=0.005
  Transport Delay1 : TransportDelay  DelayTime=0.005
  gasToForce(180=1m/ss) : MATLABFcn  MATLABFcn=gasToForce
  F : Outport
  M : Outport  Port=2
  wires:
  ROLL/1 -> Gain3/1
  NICK/1 -> Gain2/1
  YAW/1 -> Gain1/1
  Mux/1 -> Transport Delay/1
  Mux1/1 -> Transport Delay1/1
  Gain1/1 -> Add1/1
  Add1/1 -> Mux1/2
  Constant/1 -> Mux1/3, Mux1/1
  Vb/1 -> Demux1/1
  Gain2/1 -> Add2/1
  Demux1/1 -> Add2/2
  Add2/1 -> Mux/1
  Add3/1 -> Mux/3
  Demux1/3 -> Add3/2
  Gain3/1 -> Add3/1
  Transport Delay/1 -> Force/1, F/1
  Transport Delay1/1 -> M/1
  GAS/1 -> gasToForce(180=1m/ss)/1
  gasToForce(180=1m/ss)/1 -> Mux/2, Force1/1
  rad/s/1 -> Selector2/1
  Selector2/1 -> Add1/2
  Demux1/2 -> Terminator/1

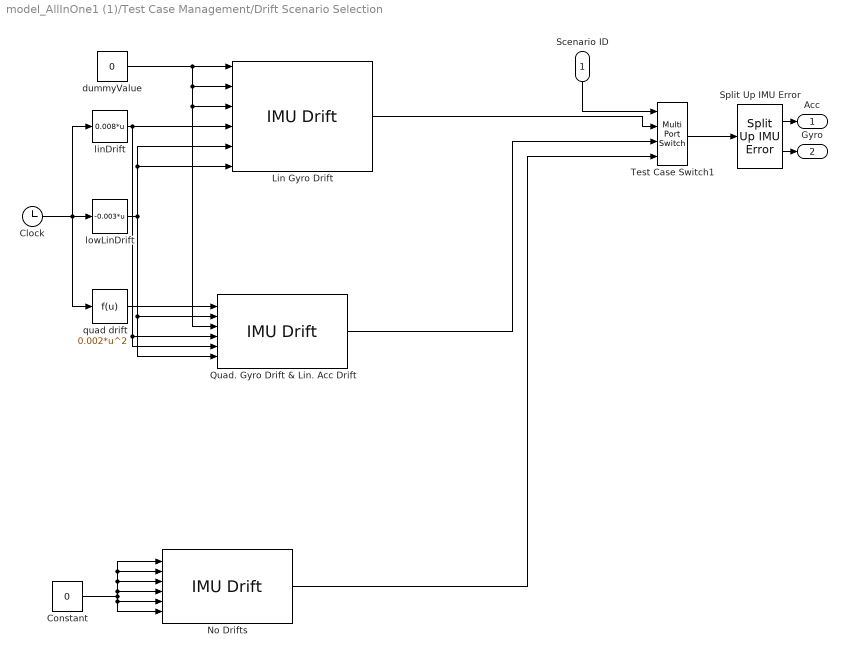
== system model_AllInOne1 (1)/Test Case Management/Drift Scenario Selection ==
  Scenario ID : Inport
  " Test Case Switch1" : MultiPortSwitch
  Clock : Clock
  Constant : Constant  Value=0
  Lin Gyro Drift : test_library/IMU Drift  SystemSampleTime=-1
  No Drifts : test_library/IMU Drift  SystemSampleTime=-1
  Quad. Gyro Drift & Lin. Acc Drift : test_library/IMU Drift  SystemSampleTime=-1
  Split Up IMU Error : test_library/Split Up IMU Error
  dummyValue : Constant  Value=0
  linDrift : Fcn  Expr=0.008*u
  lowLinDrift : Fcn  Expr=-0.003*u
  quad drift : Fcn  Expr=0.002*u^2
  Acc : Outport
  Gyro : Outport  Port=2
  wires:
  Lin Gyro Drift/1 -> " Test Case Switch1"/2
  lowLinDrift/1 -> Lin Gyro Drift/5, Lin Gyro Drift/6, Quad. Gyro Drift & Lin. Acc Drift/6, Quad. Gyro Drift & Lin. Acc Drift/2
  linDrift/1 -> Lin Gyro Drift/4, Quad. Gyro Drift & Lin. Acc Drift/1
  Clock/1 -> lowLinDrift/1, linDrift/1, quad drift/1
  Scenario ID/1 -> " Test Case Switch1"/1
  Split Up IMU Error/1 -> Acc/1
  Split Up IMU Error/2 -> Gyro/1
  quad drift/1 -> Quad. Gyro Drift & Lin. Acc Drift/4, Quad. Gyro Drift & Lin. Acc Drift/5
  " Test Case Switch1"/1 -> Split Up IMU Error/1
  No Drifts/1 -> " Test Case Switch1"/4
  Quad. Gyro Drift & Lin. Acc Drift/1 -> " Test Case Switch1"/3
  Constant/1 -> No Drifts/1, No Drifts/2, No Drifts/3, No Drifts/4, No Drifts/5, No Drifts/6
  dummyValue/1 -> Lin Gyro Drift/1, Lin Gyro Drift/2, Lin Gyro Drift/3, Quad. Gyro Drift & Lin. Acc Drift/3

== system model_AllInOne1 (1)/Test Case Management/IMU Noise Scenario Selection ==
  Scenario ID : Inport
  " Test Case Switch" : MultiPortSwitch  Inputs=4
  Hight Noise Level : test_library/IMU Noise  accX=0.1  accY=0  accZ=0.1  gX=0  gY=0  gZ=0  sTime=0.01
  Low Noise Level : test_library/IMU Noise  accX=0  accY=0.05  accZ=0  gX=0  gY=0  gZ=0  sTime=0.01
  No Noise : test_library/IMU Noise  accX=0  accY=0  accZ=0  gX=0  gY=0  gZ=0  sTime=0.01
  Split Up IMU Error : test_library/Split Up IMU Error
  Very Low Y-Noise : test_library/IMU Noise  accX=0  accY=0.025  accZ=0  gX=0  gY=0  gZ=0  sTime=0.01
  acc_noise : Outport
  gyro_noise : Outport  Port=2
  wires:
  Low Noise Level/1 -> " Test Case Switch"/2
  Hight Noise Level/1 -> " Test Case Switch"/3
  " Test Case Switch"/1 -> Split Up IMU Error/1
  Split Up IMU Error/1 -> acc_noise/1
  Split Up IMU Error/2 -> gyro_noise/1
  Scenario ID/1 -> " Test Case Switch"/1
  No Noise/1 -> " Test Case Switch"/4
  Very Low Y-Noise/1 -> " Test Case Switch"/5

== system model_AllInOne1 (1)/Test Case Management/Obstacle Scenario Management ==
  Scneario ID : Inport
  Box1 : test_library/Box  t=11  p=[42, 2, 0]  d=[1, 2, 3]  tc_ids=[1 3]
  Cube : test_library/Box  t=15  p=[0, 0, 0]  d=[1, 2, 3]  tc_ids=[2]
  Small Box : test_library/Box  t=25  p=[0, 0, 0]  d=[1, 2, 3]  tc_ids=[3]
  Vector Concatenate : Concatenate  NumInputs=3  Mode=Multidimensional array
  Obj. : Outport
  wires:
  Box1/1 -> Vector Concatenate/1
  Cube/1 -> Vector Concatenate/2
  Small Box/1 -> Vector Concatenate/3
  Scneario ID/1 -> Small Box/1, Cube/1, Box1/1
  Vector Concatenate/1 -> Obj./1

== system model_AllInOne1 (1)/Test Case Management/Sensor Blackout Scenario Selection ==
  Scenario ID : Inport
  AHRS : test_library/Blackout Scenario  tAHRS=55  tPMD=-1  tUS_GND=-1  tUS_FRONT=-1  tUS_LHS=-1  tUS_RHS=-1  tUS_CEIL=-1  tUS_REAR=-1
  Bus Selector : BusSelector  OutputSignals=bo_ahrs,bo_pmd,bo_us
  Multiport Switch : MultiPortSwitch
  No Blackout : test_library/Blackout Scenario  tAHRS=-1  tPMD=-1  tUS_GND=-1  tUS_FRONT=-1  tUS_LHS=-1  tUS_RHS=-1  tUS_CEIL=-1  tUS_REAR=-1
  PMD & UltraSonic LHS : test_library/Blackout Scenario  tAHRS=-1  tPMD=60  tUS_GND=-1  tUS_FRONT=-1  tUS_LHS=96  tUS_RHS=-1  tUS_CEIL=-1  tUS_REAR=-1
  BoAHRS : Outport
  BoPMD : Outport  Port=2
  BoUS : Outport  Port=3
  wires:
  Scenario ID/1 -> Multiport Switch/1
  AHRS/1 -> Multiport Switch/2
  PMD & UltraSonic LHS/1 -> Multiport Switch/3
  Multiport Switch/1 -> Bus Selector/1
  Bus Selector/1 -> BoAHRS/1  "<bo_ahrs>"
  Bus Selector/2 -> BoPMD/1  "<bo_pmd>"
  Bus Selector/3 -> BoUS/1  "<bo_us>"
  No Blackout/1 -> Multiport Switch/4

== system model_AllInOne1 (1)/Visualization/Plot PMD Cam Image ==
  In1 : Inport
  Data Type Conversion : DataTypeConversion
  Plot 3dCam image : MATLABFcn  MATLABFcn=plot3dCamPic  OutputDimensions=0
  Reshape : Reshape  OutputDimensionality=Customize  OutputDimensions=[48,64]
  wires:
  In1/1 -> Reshape/1
  Reshape/1 -> Data Type Conversion/1
  Data Type Conversion/1 -> Plot 3dCam image/1

== system model_AllInOne1 (1)/Visualization/Rotation ==
  phi theta psi 3x1 : Inport
  -90 degreee : Constant  Value=-1.57
  Add1 : Sum
  Demux : Demux  Outputs=3
  Mux : Mux  Inputs=2
  Mux1 : Mux  Inputs=2
  Terminator : Terminator
  Terminator1 : Terminator
  y-axis : Constant  Value=[0 1 0]
  falter rotation : Outport
  faltercamera rotation : Outport  Port=2
  wires:
  Mux/1 -> falter rotation/1
  phi theta psi 3x1/1 -> Demux/1
  y-axis/1 -> Mux/1, Mux1/1
  Demux/2 -> Add1/1, Mux/2
  -90 degreee/1 -> Add1/2
  Demux/1 -> Terminator/1
  Demux/3 -> Terminator1/1
  Mux1/1 -> faltercamera rotation/1
  Add1/1 -> Mux1/2

== system model_AllInOne1 (1)/Physical Model/6DoF (Euler Angles), incl. gravity and ground detection/Determine Force, Mass and Inertia ==
  forces : Inport
  Constant : Constant  Value=mass_0  OutDataTypeStr=Inherit: Inherit via back propagation
  Constant1 : Constant  Value=[inertia; zeros(3,3)]  OutDataTypeStr=Inherit: Inherit via back propagation
  "forces " : Outport
  mass : Outport  Port=2
  "inertia, 0" : Outport  Port=3
  wires:
  forces/1 -> "forces "/1
  Constant1/1 -> "inertia, 0"/1
  Constant/1 -> mass/1

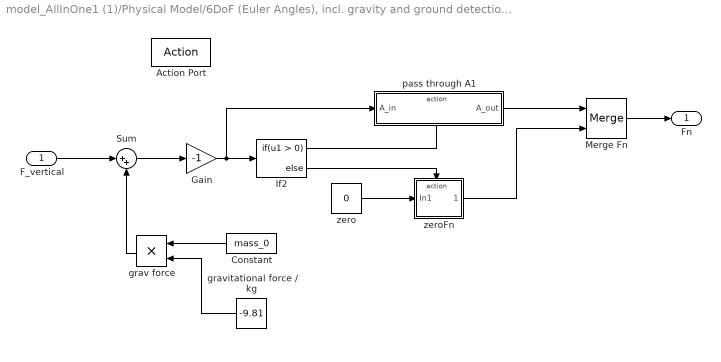
== system model_AllInOne1 (1)/Physical Model/6DoF (Euler Angles), incl. gravity and ground detection/gte zero only ==
  F_vertical : Inport
  Action Port : ActionPort  ActionType=else
  Constant : Constant  Value=mass_0  OutDataTypeStr=Inherit: Inherit via back propagation
  Gain : Gain  Gain=-1
  If2 : If
  Merge Fn : Merge
  Sum : Sum  Inputs=|++
  grav force : Product  RndMeth=Zero
  gravitational force / kg : Constant  Value=-9.81
  pass through A1 : Subsystem  TreatAsAtomicUnit=on
  zero : Constant  Value=0
  zeroFn : Subsystem  TreatAsAtomicUnit=on
  Fn : Outport
  wires:
  gravitational force / kg/1 -> grav force/2
  Constant/1 -> grav force/1
  F_vertical/1 -> Sum/1
  grav force/1 -> Sum/2
  Sum/1 -> Gain/1
  Gain/1 -> If2/1, pass through A1/1(A_in)
  If2/1 -> pass through A1/Action
  If2/2 -> zeroFn/Action
  pass through A1/1(A_out) -> Merge Fn/1
  zeroFn/1(zero_Fn) -> Merge Fn/2
  Merge Fn/1 -> Fn/1
  zero/1 -> zeroFn/1(In1)
